simulink model "SimlinkFinal"  (R2019a)
settings: Solver=VariableStepAuto  StartTime=0.0  StopTime=5  RelTol=1e-3
values from neighbouring files (symbols this model uses):
  B = 0.003    [Final.m]    (also in workspace.mat)
  Ba = 4.32e-3    (= 0.00432)    [Final.m]    (also in workspace.mat)
  J = 4.321e-4    (= 0.0004321)    [Final.m]    (also in workspace.mat)
  Ja = 2.7e-4    (= 0.00027)    [Final.m]    (also in workspace.mat)
  Kb = 0.27    [Final.m]    (also in workspace.mat)
  Kt = 0.27    [Final.m]    (also in workspace.mat)
  potentiometer = 1    [workspace.mat]
  Ra = 1.05    [Final.m]    (also in workspace.mat)
  Rg = 1.6e-4    (= 0.00016)    [Final.m]    (also in workspace.mat)
libraries: simulink x1
settings Model: Creator=MohamedRaafat  LastModifiedBy=MohamedRaafat

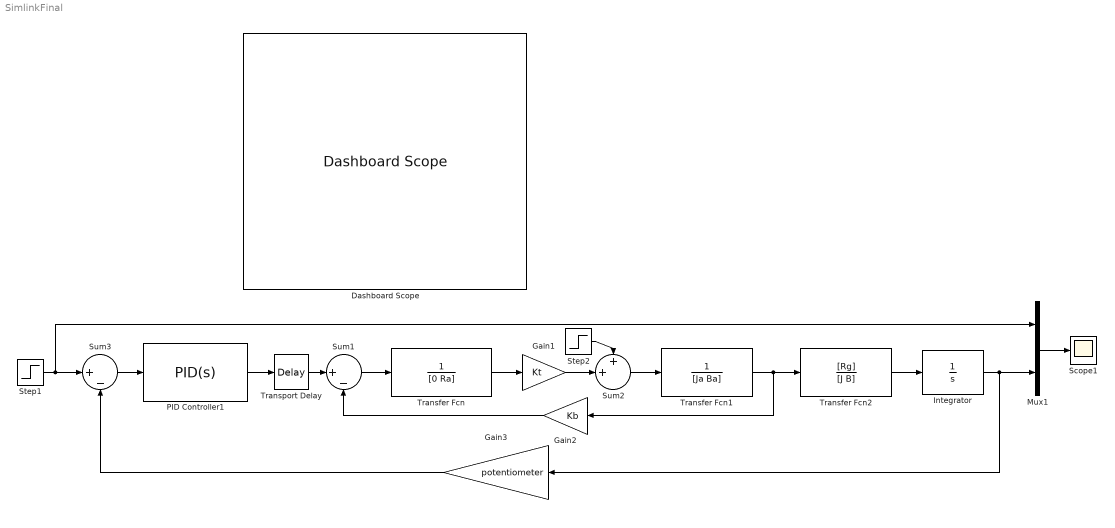
== system SimlinkFinal ==
  Dashboard Scope : DashboardScope
  Gain1 : Gain  Gain=Kt
  Gain2 : Gain  Gain=Kb
  Gain3 : Gain  Gain=potentiometer
  Integrator : Integrator
  Mux1 : Mux  Inputs=2
  PID Controller1 : simulink/Continuous/PID Controller  Controller=PID  Form=Parallel  TimeDomain=Continuous-time  SampleTime=-1  IntegratorMethod=Forward Euler  FilterMethod=Forward Euler  ControllerParametersSource=internal  P=283.729103372597  I=127.216062236304  D=43.5485225514386  UseFilter=on  N=580.71860464414  TunerSelectOption=Transfer Function Based (PID Tuner App)  InitialConditionSource=internal  InitialConditionForIntegrator=0  InitialConditionForFilter=0  DifferentiatorICPrevScaledInput=0  ExternalReset=none  TrackingMode=off  Kt=1  LimitOutput=off  UpperSaturationLimit=inf  LowerSaturationLimit=-inf  LinearizeAsGain=on  AntiWindupMode=none  Kb=1  POutMin=[]  POutMax=[]  IOutMin=[]  IOutMax=[]  DOutMin=[]  DOutMax=[]  NOutMin=[]  NOutMax=[]  SumOutMin=[]  SumOutMax=[]  SaturationOutMin=[]  SaturationOutMax=[]  PParamMin=[]  PParamMax=[]  IParamMin=[]  IParamMax=[]  DParamMin=[]  DParamMax=[]  NParamMin=[]  NParamMax=[]  KbParamMin=[]  KbParamMax=[]  KtParamMin=[]  KtParamMax=[]  KbOutMin=[]  KbOutMax=[]  KtOutMin=[]  KtOutMax=[]  IntegratorOutMin=[]  IntegratorOutMax=[]  FilterOutMin=[]  FilterOutMax=[]  SumI1OutMin=[]  SumI1OutMax=[]  SumI2OutMin=[]  SumI2OutMax=[]  SumI3OutMin=[]  SumI3OutMax=[]  SumI4OutMin=[]  SumI4OutMax=[]  SumDOutMin=[]  SumDOutMax=[]  DifferentiatorOutMin=[]  DifferentiatorOutMax=[]  FilterDiffOutCoefMin=[]  FilterDiffOutCoefMax=[]  ReciprocalOutMin=[]  ReciprocalOutMax=[]  SumDenOutMin=[]  SumDenOutMax=[]  SumNumOutMin=[]  SumNumOutMax=[]  DivideOutMin=[]  DivideOutMax=[]  IntegratorContinuousStateAttributes=''  IntegratorStateMustResolveToSignalObject=off  IntegratorRTWStateStorageClass=Auto  FilterContinuousStateAttributes=''  FilterStateMustResolveToSignalObject=off  FilterRTWStateStorageClass=Auto  ParallelPVariant=InternalParameters  IdealPVariant=Disabled  IVariant=InternalParameters  DVariant=InternalParameters  IntegratorVariant=Continuous  SatVariant=Disabled  AWVariant=Passthrough  PCopyVariant=Disabled  TRVariant=Disabled  FdbkBlocksVariant=Forward  IdealPFdbkVariant=Disabled  SatFdbkVariant=Disabled  DerivativeFilterVariant=ContFilter  NVariant=InternalParameters  NCopyVariant=Disabled  FilterICVariant=InternalICsFilter  IntegratorICVariant=InternalICs  ExternalResetVariant=Disabled  TRSumVariant=Passthrough  SumFdbkVariant=Disabled  SumVariant=Sum_PID
  Scope1 : Scope
  Step1 : Step  SampleTime=0
  Step2 : Step  SampleTime=0
  Sum1 : Sum  Inputs=|+-
  Sum2 : Sum  Inputs=++|
  Sum3 : Sum  Inputs=|+-
  Transfer Fcn : TransferFcn  Denominator=[0 Ra]
  Transfer Fcn1 : TransferFcn  Denominator=[Ja Ba]
  Transfer Fcn2 : TransferFcn  Numerator=[Rg]  Denominator=[J B]
  Transport Delay : TransportDelay  DelayTime=0
  wires:
  Transfer Fcn1/1 -> Gain2/1, Transfer Fcn2/1
  Gain2/1 -> Sum1/2
  Sum1/1 -> Transfer Fcn/1
  Mux1/1 -> Scope1/1
  PID Controller1/1 -> Transport Delay/1
  Step1/1 -> Sum3/1, Mux1/1
  Transfer Fcn/1 -> Gain1/1
  Step2/1 -> Sum2/1
  Transfer Fcn2/1 -> Integrator/1
  Gain3/1 -> Sum3/2
  Sum3/1 -> PID Controller1/1
  Integrator/1 -> Mux1/2, Gain3/1
  Transport Delay/1 -> Sum1/1
  Sum2/1 -> Transfer Fcn1/1
  Gain1/1 -> Sum2/2
